simulink model "test_topcampsi"  (R2014b)
settings: Solver=ode45  StartTime=0.0  StopTime=inf  RelTol=1e-3
InitFcn:
  | load background
  | 
  | load template_drones1
values from neighbouring files (symbols this model uses):
  backim = [6 7 7 8 8 10 12 11 11 12 13 13 ... (6220800 elements, 1080x1920x3)]    [background.mat]    (also in backgroundwebcam.mat = [186 204 204 200 195 195 195 197 194 196 199 186 ... (921600; updateBackim.m = snapshot(cam))
  C = zeros(N,2)    [psi_topviewcam_wrapped.m]
  drone1 = [0 0 1 2 3 5 6 6 7 7 7 7 ... (3828 elements, 58x22x3)]    [template_drones1.mat]
undefined symbols (not defined in the file or in its folder): DeviceSpecific, IsPositionTracked, IsSkeletonTracked, JointDepthIndices, JointImageIndices, JointTrackingState, JointWorldCoordinates, PositionDepthIndices, PositionImageIndices, PositionWorldCoordinates, SegmentationData, SkeletonTrackingID, videoinput
libraries: imaqlib x1
settings Model: Creator=s139462  LastModifiedBy=s139462
settings DataIOCC: ExternalInput=[t,u]

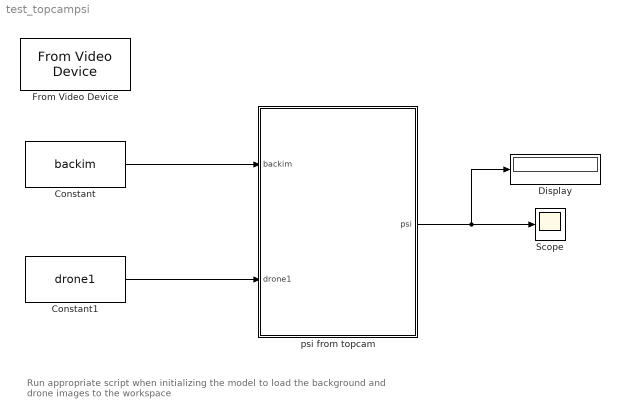
== system test_topcampsi ==
  note: Run appropriate script when initializing the model to load
      | the background and drone images to the workspace
  Constant : Constant  Value=backim
  Constant1 : Constant  Value=drone1
  Display : Display
  From Video Device : imaqlib/From Video Device  DeviceMenu=gige 1 (GE1900C (02-2081A))  Device=gige 1 (GE1900C (02-2081A))  ObjConstructor=videoinput('gige', 1)  VideoFormatMenu=Mono8  VideoFormat=Mono8  VideoSource=input1  ROIPosition=[0 0 1080 1920]  EnableHWTrigger=off  TriggerConfiguration=DeviceSpecific/DeviceSpecific  SampleTime=1/30  OutputPortsMode=One multidimensional signal  DataType=single  CanDoHWTrigger=yes  ReturnedColorSpace=rgb  BlockHandle=1921.0006  ROIWidth=640  ROIHeight=480  ROIColumn=0  ROIRow=0  EngXMLPath=C:\Program Files\MATLAB\R2014b\toolbox\imaq\imaq\private  DevXMLPath=C:\MATLAB\SupportPackages\R2014b\gigevisionhardware\toolbox\imaq\supportpackages\gige\adaptor\win64  EngLibPath=C:\Program Files\MATLAB\R2014b\toolbox\imaq\imaqblks\imaqmex\win64  ColorSpace=rgb  BayerSensorAlignment=grbg  AllMetadata=IsPositionTracked;IsSkeletonTracked;JointDepthIndices;JointImageIndices;JointTrackingState;JointWorldCoordinates;PositionDepthIndices;PositionImageIndices;PositionWorldCoordinates;SegmentationData;SkeletonTrackingID
  Scope : Scope
  psi from topcam : MATLAB Function  TreatAsAtomicUnit=on
  wires:
  psi from topcam/1(psi) -> Display/1, Scope/1
  Constant/1 -> psi from topcam/1(backim)
  Constant1/1 -> psi from topcam/2(drone1)

== matlab function test_topcampsi/psi from topcam ==
  data: backim input; psi output; drone1 input
function psi = fcn(backim, drone1)
%% get psi angle from top camera
% this function is the improcdrones.m implemented for ONLY ONE DRONE and 
% therefore reduced.




coder.extrinsic('psi_topviewcam_wrapped')
    
    psi = 0;
    psi = psi_topviewcam_wrapped(backim, drone1);

end
